simulink model "Simulink_to_xppu"  (R2020a)
settings: Solver=FixedStepDiscrete  StartTime=0.0  StopTime=10.0  FixedStep=0.1  RelTol=1e-3  EnableMultiTasking=on
settings Model: Creator=Leonardo Igler  LastModifiedBy=Leonardo Igler
settings SolverCC: AutoInsertRateTranBlk=on
settings DataIOCC: LimitDataPoints=on
settings OptimizationCC: DefaultParameterBehavior=Inlined  EnhancedBackFolding=on  PassReuseOutputArgsAs=Individual arguments  ZeroExternalMemoryAtStartup=off  ZeroInternalMemoryAtStartup=off  OptimizeBlockOrder=speed  DifferentSizesBufferReuse=on  OptimizationCustomize=off  EfficientTunableParamExpr=on
settings DebuggingCC: ParameterTunabilityLossMsg=error  AllowSymbolicDim=off  SFUnexpectedBacktrackingDiag=warning  SFNoUnconditionalDefaultTransitionDiag=warning  SFExecutionAtInitializationDiag=none  ArithmeticOperatorsInVariantConditions=warning
settings SFSimCC: SimUseLocalCustomCode=off  MATLABDynamicMemAlloc=off  CustomCodeUndefinedFunction=UseInterfaceOnly
settings RTWCC: SystemTargetFile=ert.tlc  GenCodeOnly=on  PackageGeneratedCodeAndArtifacts=on  PackageName=SimPLC  TemplateMakefile=ert_default_tmf  RTWUseLocalCustomCode=off
settings CodeAppCC: ForceParamTrailComments=on  IgnoreCustomStorageClasses=off  OperatorAnnotations=on  SimulinkDataObjDesc=on  SFDataObjDesc=on  InsertBlockDesc=on
settings ERTTargetCC: GenerateSampleERTMain=on  InlinedParameterPlacement=NonHierarchical  ERTCustomFileTemplate=example_file_process.tlc
settings ConfigComp: CovMetricSettings=dw  CovHtmlReporting=on  CovSaveCumulativeToWorkspaceVar=on  CovSaveSingleToWorkspaceVar=on  CovShowResultsExplorer=off  CovExternalEMLEnable=off  CovSFcnEnable=off  PLC_TargetIDE=twincat3

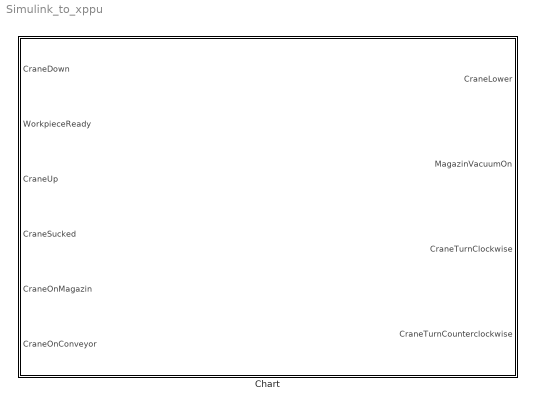
== system Simulink_to_xppu ==
  Chart : Stateflow chart  TreatAsAtomicUnit=on

== stateflow chart Simulink_to_xppu/Chart ==
  state Start
    entry:
    CraneLower = false;
    MagazinVacuumOn = false;
    CraneTurnCounterclockwise = false;
    CraneTurnClockwise = false;
  state Initializing1
    entry:
    CraneLower =true ;
  state Initializing2
    entry:
    CraneLower = false;
  state Lookinf_for_WP
  state Crane_Rightturn
    during:
    CraneTurnClockwise = true;
    CraneTurnCounterclockwise = false;
  state At_Magazine
    CraneTurnClockwise = false;
    CraneTurnCounterclockwise =false ;
  state Crane_Down
    MagazinVacuumOn = true;
    CraneLower = true;;
  state Crane_Up
    during:
    CraneLower = false;
  state Crane_Leftturn
    during:
    CraneTurnCounterclockwise = true;
    CraneTurnClockwise = false;
  state Crane_at_Conveyor
    during:
    CraneTurnCounterclockwise = false;
    CraneTurnClockwise = false;
    CraneLower = true;
  state Lei_it_go
    during:
    MagazinVacuumOn = false;
  state Up_again
    during:
    CraneLower = false;
  state DONE
  (default) -> Start
  Start -> Initializing1 : [true]
  Initializing1 -> Initializing2 : [CraneDown]
  Initializing2 -> Lookinf_for_WP : [CraneUp]
  DONE -> Lookinf_for_WP : [true]
  Lookinf_for_WP -> Crane_Rightturn : [WorkpieceReady==true]
  Crane_Rightturn -> At_Magazine : [CraneOnMagazin]
  At_Magazine -> Crane_Down : [true]
  Crane_Down -> Crane_Up : [CraneSucked]
  Crane_Up -> Crane_Leftturn : [CraneUp]
  Crane_Leftturn -> Crane_at_Conveyor : [CraneOnConveyor]
  Crane_at_Conveyor -> Lei_it_go : [CraneDown]
  Lei_it_go -> Up_again : [true]
  Up_again -> DONE : [CraneUp]
  data: CraneDown input boolean; WorkpieceReady input boolean; CraneLower output boolean; MagazinVacuumOn output boolean; CraneUp input boolean; CraneSucked input boolean; CraneOnMagazin input boolean; CraneTurnClockwise output boolean; CraneTurnCounterclockwise output boolean; CraneOnConveyor input boolean
